simulink model "vessel"  (R2022a)
settings: Solver=ode4  StartTime=0.0  StopTime=50  FixedStep=0.01  RelTol=1e-3
values from neighbouring files (symbols this model uses):
  initial_pose = [0,0,0,0,0,0]'    [init_vessel.m]
  initial_velocity = [0,0,0,0,0,0]'    [init_vessel.m]
libraries: mssSimulink x5
settings Model: Creator=tobiasvt  LastModifiedBy=HalvorPlatou
settings SolverCC: AlgebraicLoopSolver=TrustRegion
settings DebuggingCC: UnconnectedInputMsg=warning  UnconnectedOutputMsg=warning  UnconnectedLineMsg=warning  SFMachineParentedDataDiag=warning
settings SFSimCC: CustomCodeUndefinedFunction=UseInterfaceOnly
settings RTWCC: Description=FMU based on GRT (Functional Mock-up Unit)  SystemTargetFile=grtfmi.tlc  GenerateMakefile=off  TemplateMakefile=none  RetainRTWFile=on
settings STFCustomTargetCC: TargetLangStandard=C99 (ISO)  CombineOutputUpdateFcns=on  CodeInterfacePackaging=Reusable function  GRTInterface=off  GenerateAllocFcn=on  SystemTargetFile=grtfmi.tlc
settings GRTTargetCC: ParMdlRefBuildCompliant=off  CompOptLevelCompliant=off  ConcurrentExecutionCompliant=off  MatFileLogging=off  CodeInterfacePackaging=Reusable function  CPPClassGenCompliant=off  GenerateAllocFcn=on  UseToolchainInfoCompliant=off

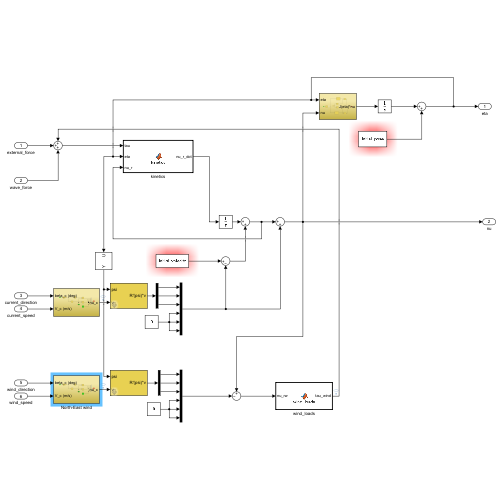
[thumbnail: Simulink's stored preview of the top-level diagram]
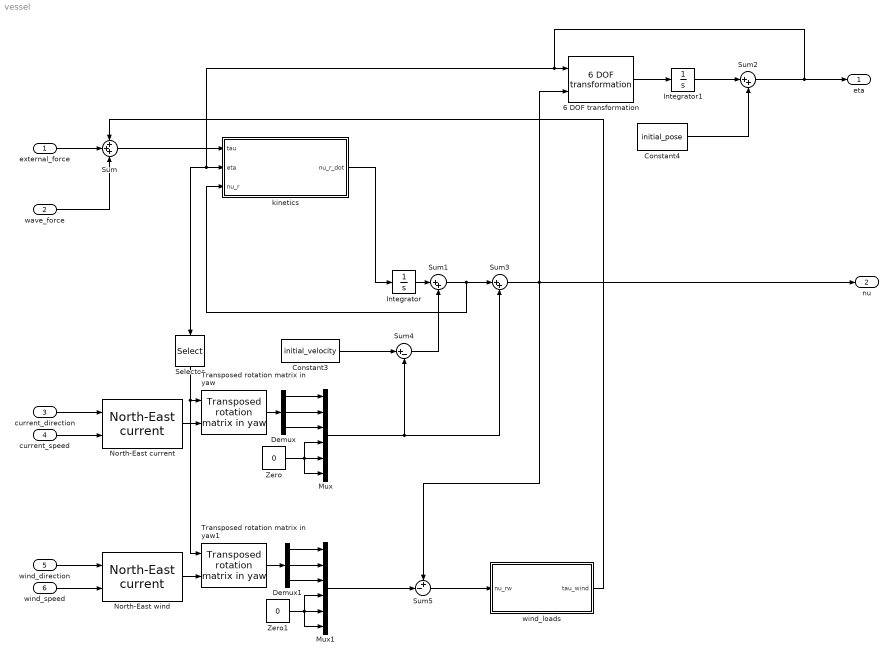
== system vessel ==
  external_force : Inport  PortDimensions=6
  wave_force : Inport  Port=2  PortDimensions=6
  current_direction : Inport  Port=3  PortDimensions=1
  current_speed : Inport  Port=4  PortDimensions=1
  wind_direction : Inport  Port=5  PortDimensions=1
  wind_speed : Inport  Port=6  PortDimensions=1
  6 DOF transformation : mssSimulink/Modelling/Kinematics/6 DOF transformation  SystemSampleTime=-1  VariantActivationTime=update diagram  Latency=0  AutoFrameSizeCalculation=off
  Constant3 : Constant  Value=initial_velocity
  Constant4 : Constant  Value=initial_pose
  Demux : Demux  Outputs=3
  Demux1 : Demux  Outputs=3
  Integrator : Integrator
  Integrator1 : Integrator
  Mux : Mux  Inputs=6
  Mux1 : Mux  Inputs=6
  North-East current : mssSimulink/Environment/Current/North-East current  SystemSampleTime=-1  VariantActivationTime=update diagram  Latency=0  AutoFrameSizeCalculation=off
  North-East wind : mssSimulink/Environment/Current/North-East current  SystemSampleTime=-1  VariantActivationTime=update diagram  Latency=0  AutoFrameSizeCalculation=off
  Selector : Selector  InputPortWidth=6  IndexOptions=Index vector (dialog)  Indices=[6]  OutputSizes=1
  Sum : Sum  Inputs=+++
  Sum1 : Sum  Inputs=|++
  Sum2 : Sum  Inputs=|++
  Sum3 : Sum  Inputs=|++
  Sum4 : Sum  Inputs=|+-
  Sum5 : Sum  Inputs=+-|
  Transposed rotation matrix in yaw : mssSimulink/Modelling/Kinematics/Transposed rotation  matrix in yaw
  Transposed rotation matrix in yaw1 : mssSimulink/Modelling/Kinematics/Transposed rotation  matrix in yaw
  Zero : Constant  Value=0  OutDataTypeStr=Inherit: Inherit via back propagation
  Zero1 : Constant  Value=0  OutDataTypeStr=Inherit: Inherit via back propagation
  kinetics : MATLAB Function  TreatAsAtomicUnit=on
  wind_loads : MATLAB Function  TreatAsAtomicUnit=on
  eta : Outport  VectorParamsAs1DForOutWhenUnconnected=off
  nu : Outport  Port=2  VectorParamsAs1DForOutWhenUnconnected=off
  wires:
  Demux1/1 -> Mux1/1
  North-East wind/1 -> Transposed rotation matrix in yaw1/2
  Mux1/1 -> Sum5/2
  Transposed rotation matrix in yaw1/1 -> Demux1/1
  Zero1/1 -> Mux1/6, Mux1/4, Mux1/5
  Demux/1 -> Mux/1
  Sum1/1 -> kinetics/3(nu_r), Sum3/1
  Demux1/2 -> Mux1/2
  wind_direction/1 -> North-East wind/1
  Demux/3 -> Mux/3
  Sum5/1 -> wind_loads/1(nu_rw)
  Demux1/3 -> Mux1/3
  North-East current/1 -> Transposed rotation matrix in yaw/2
  Sum2/1 -> kinetics/2(eta), Selector/1, 6 DOF transformation/1, eta/1
  Mux/1 -> Sum4/2, Sum3/2
  external_force/1 -> Sum/2
  Demux/2 -> Mux/2
  kinetics/1(nu_r_dot) -> Integrator/1
  Transposed rotation matrix in yaw/1 -> Demux/1
  Integrator/1 -> Sum1/1
  Zero/1 -> Mux/6, Mux/4, Mux/5
  Constant4/1 -> Sum2/2
  Sum3/1 -> Sum5/1, 6 DOF transformation/2, nu/1
  current_speed/1 -> North-East current/2
  Selector/1 -> Transposed rotation matrix in yaw1/1, Transposed rotation matrix in yaw/1
  Sum/1 -> kinetics/1(tau)
  wave_force/1 -> Sum/3
  Integrator1/1 -> Sum2/1
  Constant3/1 -> Sum4/1
  Sum4/1 -> Sum1/2
  wind_speed/1 -> North-East wind/2
  current_direction/1 -> North-East current/1
  6 DOF transformation/1 -> Integrator1/1
  wind_loads/1(tau_wind) -> Sum/1

== matlab function vessel/wind_loads ==
  data: nu_rw input; tau_wind output
function tau_wind = wind_loads(nu_rw)
    gamma_rw = -atan2(nu_rw(2),nu_rw(1));
    V_rw = sqrt(nu_rw(1)^2 + nu_rw(2)^2);
    rho_a = 1.225;
    
    
    % Blendermann (1994) Wind load model based on data from Anders Pedersen (2019)
    A_Fw = 2.9;
    A_Lw = 8.6;
    L_oa = 5.0;
    s_L = 0.0;
    H_Lw = 1.0;
    delta = 0.8;
    kappa = 1.1;
    CD_t = 0.9;
    CD_lAF = 0.475;
    CD_l = CD_lAF*A_Fw/A_Lw;
    
    C_X = -CD_lAF*(cos(gamma_rw))/(1-0.5*delta*(1-(CD_l/CD_t))*sin(2*gamma_rw)^2);
    C_Y = CD_t*(sin(gamma_rw))/(1-0.5*delta*(1-(CD_l/CD_t))*sin(2*gamma_rw)^2);
    C_K = kappa*C_Y;
    C_N = ((s_L/L_oa) - 0.18*(abs(gamma_rw)-0.5*pi))*C_Y;
    
    tau_wind = 0.5*rho_a*V_rw^2*[C_X*A_Fw;
                                 C_Y*A_Lw;
                                 0.0;
                                 C_K*A_Lw*H_Lw;
                                 0.0;
                                 C_N*A_Lw*L_oa];
end

== matlab function vessel/kinetics ==
  data: tau input; eta input; nu_r_dot output; nu_r input
function nu_r_dot = kinetics(tau, eta, nu_r)
    %% Horizontal kinetics
    %Hydrodynamic coefficients
    m_11 = 2390;
    m_12 = 0.0;
    m_13 = 0.0;
    m_21 = 0.0;
    m_22 = 2448;
    m_23 = 268.1;
    m_31 = 0.0;
    m_32 = -23.84;
    m_33 = 4862;
    X_u = -106.6;
    X_auu = -21.39;
    X_uuu = -37.43;
    X_v = 0.0;
    X_r = 0.0;
    Y_u = 0.0;
    Y_v = -29.44;
    Y_avv = -172.9;
    Y_vvv = -1.338;
    Y_arv = -1517;
    Y_r = 62.58;
    Y_avr = 488.7;
    Y_arr = -198.2;
    N_u = 0.0;
    N_v = 7.34;
    N_avv = -4.352;
    N_arv = 437.8;
    N_r = -142.7;
    N_arr = -831.7;
    N_rrr = 0;
    N_avr = -122;
    Y_ur = 77.58;
    N_uv = -90.97;
    N_ur = 178.5;
    
    u = nu_r(1);
	v = nu_r(2);
	r = nu_r(6);
    
    %Mass matrix
    M = [m_11 0.0 0.0;
         0.0 m_22 m_23;
         0.0 m_32 m_33];
     
    M_inv = inv(M);
    
    %Damping matrix
    d_11 = -X_u - X_auu*abs(u) - X_uuu*u^2;
    d_12 = -X_v;
    d_13 = -X_r;
    d_21 = -Y_u;
    d_22 = -Y_v - Y_avv*abs(v) - Y_arv*abs(r) - Y_vvv*v^2;
    d_23 = -Y_r - Y_avr*abs(v) - Y_arr*abs(r) - Y_ur*u;
    d_31 = -N_u;
    d_32 = -N_v - N_avv*abs(v) - N_arv*abs(r) - N_uv*u;
    d_33 = -N_r - N_avr*abs(v) - N_arr*abs(r) - N_ur*u;

    D = [d_11, d_12, d_13;
        d_21, d_22, d_23;
        d_31, d_32, d_33];
    
    %Coriolis matrix
    c_13 = -0.5*(m_21 + m_12)*u - m_22*v - 0.5*(m_23 + m_32)*r;
    c_23 =  m_11*u + 0.5*(m_21 + m_12)*v + 0.5*(m_13 + m_31)*r;
    c_31 = -c_13;
    c_32 = -c_23;

    C = [0, 0, c_13;
        0, 0, c_23;
        c_31, c_32, 0];
    
   nu_dot_hor = M_inv*(-(D + C)*[u,v,r]' + tau([1 2 6]));
   
   %% Vertical kinetics
   %Damping ratios
   zeta_heave = 0.1;
   zeta_roll = 0.1;
   zeta_pitch = 0.1;
   
   Zeta = diag([zeta_heave, zeta_roll, zeta_pitch]);
   
   %Natural periods
   T_heave = 1.0;
   T_roll = 1.0;
   T_pitch = 2.0;
   Omega = diag([2*pi/T_heave, 2*pi/T_roll, 2*pi/T_pitch]);
   
   %Inertias (including added mass)
   % Calculated assuming moment of inertia is for a uniform rectangle and
   % added mass = actual mass -> m_33 = 2*m, m_44 = 2*I_44, m_55 = 2*I_55
   m_33 = 3334;
   m_44 = 2356;
   m_55 = 7124;
   M_vert = diag([m_33, m_44, m_55]);
   
   nu_vert = nu_r([3,4,5]);
   eta_vert = eta([3,4,5]);
   tau_vert = tau([3,4,5]);
   
   nu_dot_vert = -2*Zeta*Omega*nu_vert - Omega^2*eta_vert + M_vert\tau_vert;
   
   
   nu_r_dot = [nu_dot_hor(1), nu_dot_hor(2) nu_dot_vert(1) ...
            nu_dot_vert(2), nu_dot_vert(3), nu_dot_hor(3)]';

end
